simulink model "DAddConAA"  (Simulink 7.8)
settings: Solver=ode45  StartTime=0.0  StopTime=10.0  RelTol=1e-3
settings Model: Creator=fkolass  LastModifiedBy=fkolass

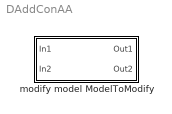
== system DAddConAA ==
  modify model ModelToModify : Subsystem

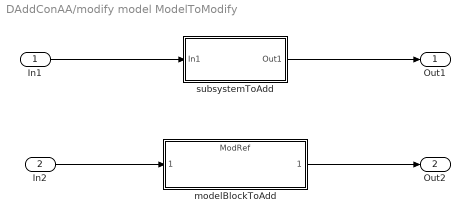
== system DAddConAA/modify model ModelToModify ==
  In1 : Inport
  In2 : Inport  Port=2
  modelBlockToAdd : ModelReference  ModelNameDialog=ModRef  SimulationMode=Normal  ModelReferenceVersion=1.2  CopyOfModelName=ModRef  DefaultDataLogging=on
  subsystemToAdd : Subsystem
  Out1 : Outport
  Out2 : Outport  Port=2
  wires:
  In1/1 -> subsystemToAdd/1(In1)
  subsystemToAdd/1(Out1) -> Out1/1
  modelBlockToAdd/1 -> Out2/1
  In2/1 -> modelBlockToAdd/1

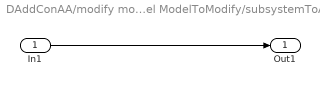
== system DAddConAA/modify model ModelToModify/subsystemToAdd ==
  In1 : Inport
  Out1 : Outport
  wires:
  In1/1 -> Out1/1
